simulink model "inverted_pendulum_model_accurate"  (R2016b)
settings: Solver=VariableStepAuto  StartTime=0.0  StopTime=100  RelTol=1e-3
values from neighbouring files (symbols this model uses):
  B = sys.B    [LoopGain.m]    (also in dcontrold_dir.m = sys_d.B; main.m = [                   0; ( 3*Km*Vs)/(LinkMass*(LinkLength^2)*R; simulation.m)
  g = 9.81    [main.m]
  Kb = Km    (= 0.0265805280355)    [main.m]
  Km = Vs/kappa_id    (= 0.0265805280355)    [main.m]    (also in sysStateEstimatorFeedbackWithModel.m = Kaug(nStates + 1:end))
  L = place(A',C',Lp)'    [dcontrold_dir.m]    (also in dcontrold_ind.m = place(A', C', desObsPoles).')
  Vs = 12    [main.m]
undefined symbols (not defined in the file or in its folder): m, R
settings Model: Creator=pong0923  LastModifiedBy=pong0923
settings DataIOCC: ExternalInput=[m]  LoadExternalInput=on

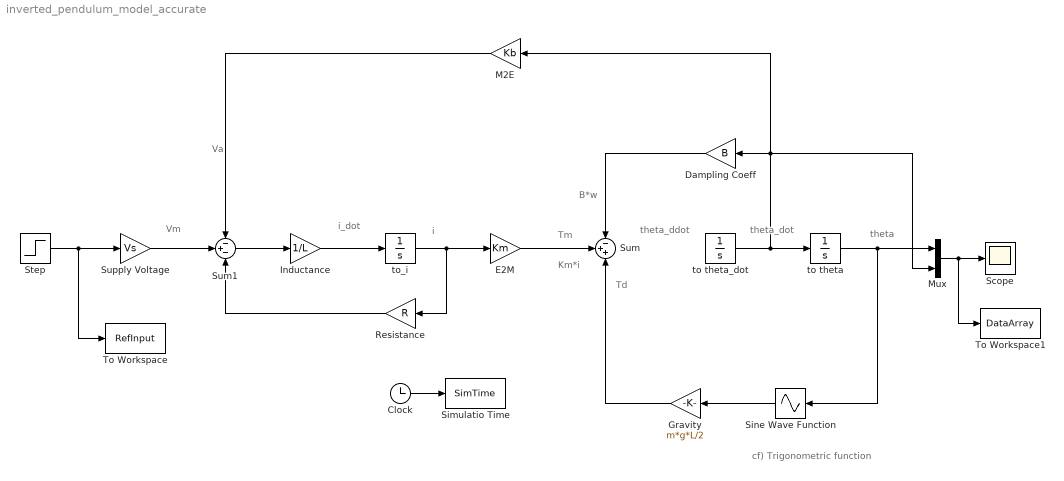
== system inverted_pendulum_model_accurate ==
  note: Va
  note: Vm
  note: i_dot
  note: B*w
  note: Td
  note: Km*i
  note: Tm
  note: i
  note: cf) Trigonometric
      | function
  note: theta_ddot
  note: theta
  note: theta_dot
  Clock : Clock
  Dampling Coeff : Gain  Gain=B
  E2M : Gain  Gain=Km
  Gravity : Gain  Gain=m*g*L/2
  Inductance : Gain  Gain=1/L
  M2E : Gain  Gain=Kb
  Mux : Mux  Inputs=2
  Resistance : Gain  Gain=R
  Scope : Scope
  Simulatio Time : ToWorkspace  VariableName=SimTime  SampleTime=-1
  Sine Wave Function : Sin  TimeSource=Use external signal  SampleTime=0
  Step : Step  After=.1  SampleTime=0
  Sum : Sum  Inputs=-++
  Sum1 : Sum  Inputs=-+-
  Supply Voltage : Gain  Gain=Vs
  To Workspace : ToWorkspace  VariableName=RefInput  SampleTime=-1
  To Workspace1 : ToWorkspace  VariableName=DataArray  SampleTime=-1
  to theta : Integrator
  to theta_dot : Integrator
  to_i : Integrator
  wires:
  to theta_dot/1 -> to theta/1, Mux/2, M2E/1, Dampling Coeff/1
  to theta/1 -> Mux/1, Sine Wave Function/1
  Sine Wave Function/1 -> Gravity/1
  E2M/1 -> Sum/2
  Dampling Coeff/1 -> Sum/1
  Gravity/1 -> Sum/3
  to_i/1 -> Resistance/1, E2M/1
  Resistance/1 -> Sum1/3
  Supply Voltage/1 -> Sum1/2
  M2E/1 -> Sum1/1
  Sum1/1 -> Inductance/1
  Inductance/1 -> to_i/1
  Step/1 -> To Workspace/1, Supply Voltage/1
  Mux/1 -> To Workspace1/1, Scope/1
  Clock/1 -> Simulatio Time/1
